simulink model "RadarSimulinkProjectRev005"  (R2024a)
settings: Solver=VariableStepAuto  StartTime=0.0  StopTime=0.0576  RelTol=1e-3
values from neighbouring files (symbols this model uses):
  AngleTime = SweepTime/10    (= 10000)    [InitializationOfVariablesRev000.m]    (also in InitializationOfVariablesRev001.m; InitializationOfVariablesRev002.m = 2000; InitializationOfVariablesRev003.m = 20000; InitializationOfVariablesRev004.m = 2097152)
  ASR_LUT = Rsamp    [InitializationOfVariablesRev003.m]    (also in InitializationOfVariablesRev004.m = round((R*2*SystemFs)/c); InitializationOfVariablesRev005.m = round((R*2*SystemFs)/c))
  Btn_Debounce = 20000    [InitializationOfVariablesRev003.m]    (also in InitializationOfVariablesRev004.m; InitializationOfVariablesRev005.m)
  ChirpNc = 128    [InitializationOfVariablesRev004.m]    (also in InitializationOfVariablesRev005.m)
  ChirpSizeLength = length(FCW)    [InitializationOfVariablesRev004.m]    (also in InitializationOfVariablesRev005.m = 16384)
  FCW = [FCW_p1, FCW_p2]    [InitializationOfVariablesRev002.m]    (also in InitializationOfVariablesRev003.m; InitializationOfVariablesRev004.m = interp1(1:length(FCW_base), FCW_base,      linspace(1, lengt; InitializationOfVariablesRev005.m = f / SystemFs)
  filt2divide = sum(h2_int)    [InitializationOfVariablesRev004.m]
  RXFFTLength = 4096    [InitializationOfVariablesRev003.m]    (also in InitializationOfVariablesRev004.m = 1024; InitializationOfVariablesRev005.m = 2048)
  SweepTime = 100000    [InitializationOfVariablesRev000.m]    (also in InitializationOfVariablesRev001.m; InitializationOfVariablesRev002.m = 20000; InitializationOfVariablesRev003.m = 200000; InitializationOfVariablesRev004.m = 23068672)
undefined symbols (not defined in the file or in its folder): SignalGenerationForAnalysis, Subsystem, xc7a200tfbg676
libraries: hdlBasic x350, hdlDSPIP x16, hdlUtilities x11, vmcUtilities x1
(part 2 of 4)

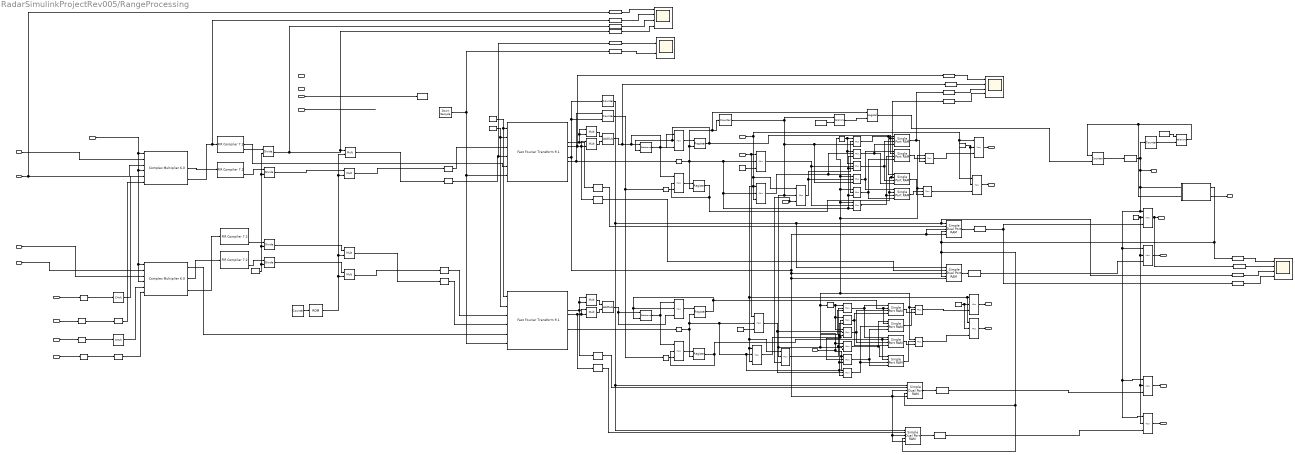
== system RadarSimulinkProjectRev005/RangeProcessing ==
  note: Tready will last until end of all 131072 samples, use for Doppler FFT
  note: These blocks are still needed for transmitting the range
  note: Will be 1 at PreDelay of EOF process, and 0 at end
      | 0 = pass through, 1 = STOP writting.
  note: Will switch to different RAM for doing the read operations, but delay not accounted
      | for the 50,000 sample delay for doppler FFT. Need to switch off WE and hold.
  note: Describes what chirp we are on, it's enable will trigger at the end of each FFT
  note: All Delays for after base Sig has been emitted
      | DDS (1) + CompMult (50) = (51)
  note: Delays per sample:
      | -Before Emittance (1)
      | -Simulated Signal (50)
      | -Recv Mixer (50)
      | -Windowing (3)
  note: TX1SimIOut
  note: TX1SimQOut
  note: TX2SimIOut
  note: TX2SimQOut
  note: TX1_REFIOut
  note: TX1_REFQOut
  note: TX2_REFIOut
  note: TX2_REFQOut
  note: Dechirp (mix with reference)
  note: Timing Assist Values (11=EOF pulse, 10=Frame Start, 9=chirp start pulse)
  note: WindowingFunction
  note: Windowing Multiplication
  note: For Syncronization: All references to frame and chirp switching need to be delayed only by the amount of delay between when it is called to toggle, and when it leaves the radar system.
      |
      | For any delay occuring within the simulation part after, this must be accounted for in the addressable shift register (delay) which simulates range delay. This delay has nothing to do with determinng when a chirp or frame has started/ended. The minimum delay, if not 0, will need to be acounted for.
      |
      | For any delay after reception, such as windowing or multiplication, this delay is relevant to anything that has to do with the processes that depend on knowing when a frame or chirp has started/ended. Since it should only start sampling once a signal theoretically should have arrived from 0 meters (no sim delay)
  note: All Delays After Dechirp
      | Delay = (101)
  note: Delay, accounting for sample missmatch
      | Delay = (104 + 139) = (243)
  note: All Delays After Window
      | Delay = (104)
  TX1SimQOut : Inport
  TX1SimIOut : Inport  Port=2
  TX2SimQOut : Inport  Port=3
  TX2SimIOut : Inport  Port=4
  TX1_REFQOut : Inport  Port=5
  TX1_REFIOut : Inport  Port=6
  TX2_REFQOut : Inport  Port=7
  TX2_REFIOut : Inport  Port=8
  BgnChirp : Inport  Port=9
  BgnFrame : Inport  Port=10
  EOChirp : Inport  Port=11
  tvalid : Inport  Port=12
  EOFDataSel : Inport  Port=13
  EOFDataAdrr : Inport  Port=14
  FlipRAM : Inport  Port=15
  PreDelayWEDisable : Inport  Port=16
  Middleofchirp : Inport  Port=17
  ADDRSwitch{,1..3} (4 alike) : hdlBasic/Mux  inputs=2  en=off  latency=0  precision=Full  arith_type=Unsigned  n_bits=16  bin_pt=14  quantization=Truncate  overflow=Wrap  XmcBlockStatus=1  maskContainerNames=tabcontainer1  block_type=mux  block_config=sysgen:Mux_config
  AddSub : hdlBasic/AddSub  mode=Addition  use_carryin=off  use_carryout=off  en=off  latency=0  precision=Full  arith_type=Unsigned  n_bits=16  bin_pt=14  quantization=Truncate  overflow=Wrap  use_behavioral_HDL=off  hw_selection=Fabric  pipelined=off  XmcBlockStatus=1  maskContainerNames=tabcontainer1  block_type=addsub  block_config=sysgen:Addsub_config
  AddSub1 : hdlBasic/AddSub  mode=Addition  use_carryin=off  use_carryout=off  en=off  latency=0  precision=Full  arith_type=Unsigned  n_bits=16  bin_pt=14  quantization=Truncate  overflow=Wrap  use_behavioral_HDL=off  hw_selection=Fabric  pipelined=off  XmcBlockStatus=1  maskContainerNames=tabcontainer1  block_type=addsub  block_config=sysgen:Addsub_config
  AddrCountPerChirp : hdlBasic/Counter  cnt_type=Count limited  cnt_to=ChirpNc-1  operation=Up  start_count=0  cnt_by_val=1  arith_type=Unsigned  n_bits=7  bin_pt=0  load_pin=off  rst=off  en=on  explicit_period=Explicit  period=P1  use_behavioral_HDL=off  implementation=Fabric  XmcBlockStatus=1  maskContainerNames=group1  block_type=counter  block_config=sysgen:Counter_config  block_width=531  block_height=1023
  AddrforIQvals : hdlBasic/Counter  cnt_type=Count limited  cnt_to=ChirpNc*RXFFTLength-1  operation=Up  start_count=0  cnt_by_val=1  arith_type=Unsigned  n_bits=17  bin_pt=0  load_pin=off  rst=off  en=on  explicit_period=Explicit  period=P1  use_behavioral_HDL=off  implementation=Fabric  XmcBlockStatus=1  maskContainerNames=group1  block_type=counter  block_config=sysgen:Counter_config  block_width=531  block_height=1023
  CMult : hdlBasic/CMult  const=-1  gui_display_data_type=Fixed-point  const_n_bits=1  const_bin_pt=0  float_type=Single  exp_bits=8  fraction_bits=24  en=off  latency=0  precision=Full  arith_type="Signed  (2's comp)"  n_bits=16  bin_pt=14  quantization=Truncate  overflow=Wrap  use_behavioral_HDL=off  mem_type=Distributed RAM  pipeline=off  XmcBlockStatus=1  maskContainerNames=tabcontainer1  block_type=cmult  block_config=sysgen:CMult_config
      settings: infoedit=[]
  CMult1 : hdlBasic/CMult  const=-1  gui_display_data_type=Fixed-point  const_n_bits=1  const_bin_pt=0  float_type=Single  exp_bits=8  fraction_bits=24  en=off  latency=0  precision=Full  arith_type="Signed  (2's comp)"  n_bits=16  bin_pt=14  quantization=Truncate  overflow=Wrap  use_behavioral_HDL=off  mem_type=Distributed RAM  pipeline=off  XmcBlockStatus=1  maskContainerNames=tabcontainer1  block_type=cmult  block_config=sysgen:CMult_config
      settings: infoedit=[]
  ChirpSamples : hdlBasic/Constant  const=ChirpNc*RXFFTLength-1  gui_display_data_type=Fixed-point  arith_type=Unsigned  n_bits=32  bin_pt=0  preci_type=Single  exp_width=8  frac_width=24  explicit_period=on  period=P2  XmcBlockStatus=1  maskContainerNames=tabcontainer1  block_type=constant  block_config=sysgen:Constant_config
  Complex Multiplier 6.0 : hdlDSPIP/Complex Multiplier 6.0   datatype=integer  hasatlast=off  hasatuser=off  atuserwidth=1  hasbtlast=off  hasbtuser=off  btuserwidth=1  multtype=Use_Mults  optimizegoal=Resources  flowcontrol=NonBlocking  outputwidth=34  roundmode=Truncate  hasctrltlast=off  hasctrltuser=off  ctrltuserwidth=1  outtlastbehv=Null  latencyconfig=Manual  minimumlatency=50  aclken=off  aresetn=off  trim_axipin_name=on  simulation_type=hybrid_sim  simulation_model=sysgen:cmpy_v6_0  data_path_portlist={ 's_axis_a_tdata_real', 's_axis_a_tdata_imag', 's_axis_b_tdata_real', 's_axis_b_tdata_imag', 's_axis_ctrl_tdata_rounding_bit', 'm_axis_dout_tdata_real', 'm_axis_dout_tdata_imag' }  aportwidth=63  bportwidth=63  ip_name=Complex Multiplier  ip_version=6.0  dsptool_ready=true  ipcore_usecache=true  ipcore_useipmodelcache=true  ipcore_verbose=false  ipcore_latency_parameter='minimumlatency'  wrapper_available=true  port_translation_map={ 'aclken' => 'en', 'aresetn' => 'rst'}  XmcBlockStatus=1  maskContainerNames=tabcontainer1  block_type=cmpy_v6_0  block_config=sysgen:rodinimport_config
  Complex Multiplier 6.1 : hdlDSPIP/Complex Multiplier 6.0   datatype=integer  hasatlast=off  hasatuser=off  atuserwidth=1  hasbtlast=off  hasbtuser=off  btuserwidth=1  multtype=Use_Mults  optimizegoal=Resources  flowcontrol=NonBlocking  outputwidth=34  roundmode=Truncate  hasctrltlast=off  hasctrltuser=off  ctrltuserwidth=1  outtlastbehv=Null  latencyconfig=Manual  minimumlatency=50  aclken=off  aresetn=off  trim_axipin_name=on  simulation_type=hybrid_sim  simulation_model=sysgen:cmpy_v6_0  data_path_portlist={ 's_axis_a_tdata_real', 's_axis_a_tdata_imag', 's_axis_b_tdata_real', 's_axis_b_tdata_imag', 's_axis_ctrl_tdata_rounding_bit', 'm_axis_dout_tdata_real', 'm_axis_dout_tdata_imag' }  aportwidth=63  bportwidth=63  ip_name=Complex Multiplier  ip_version=6.0  dsptool_ready=true  ipcore_usecache=true  ipcore_useipmodelcache=true  ipcore_verbose=false  ipcore_latency_parameter='minimumlatency'  wrapper_available=true  port_translation_map={ 'aclken' => 'en', 'aresetn' => 'rst'}  XmcBlockStatus=1  maskContainerNames=tabcontainer1  block_type=cmpy_v6_0  block_config=sysgen:rodinimport_config
  Constant : hdlBasic/Constant  const=filt2divide  gui_display_data_type=Fixed-point  arith_type=Signed (2's comp)  n_bits=32  bin_pt=0  preci_type=Single  exp_width=8  frac_width=24  explicit_period=off  period=1/200e6  XmcBlockStatus=1  maskContainerNames=tabcontainer1  block_type=constant  block_config=sysgen:Constant_config
  Constant2 : hdlBasic/Constant  const=0  gui_display_data_type=Fixed-point  arith_type=Signed (2's comp)  n_bits=16  bin_pt=15  preci_type=Single  exp_width=8  frac_width=24  explicit_period=on  period=P2  XmcBlockStatus=1  maskContainerNames=tabcontainer1  block_type=constant  block_config=sysgen:Constant_config
  Constant4 : hdlBasic/Constant  const=0  gui_display_data_type=Boolean  arith_type=Boolean  n_bits=16  bin_pt=15  preci_type=Single  exp_width=8  frac_width=24  explicit_period=on  period=P2  XmcBlockStatus=1  maskContainerNames=tabcontainer1  block_type=constant  block_config=sysgen:Constant_config
  Constant5 : hdlBasic/Constant  const=0  gui_display_data_type=Boolean  arith_type=Boolean  n_bits=16  bin_pt=15  preci_type=Single  exp_width=8  frac_width=24  explicit_period=on  period=P2  XmcBlockStatus=1  maskContainerNames=tabcontainer1  block_type=constant  block_config=sysgen:Constant_config
  Constant6 : hdlBasic/Constant  const=0  gui_display_data_type=Fixed-point  arith_type=Signed (2's comp)  n_bits=16  bin_pt=15  preci_type=Single  exp_width=8  frac_width=24  explicit_period=on  period=P2  XmcBlockStatus=1  maskContainerNames=tabcontainer1  block_type=constant  block_config=sysgen:Constant_config
  Constant7 : hdlBasic/Constant  const=0  gui_display_data_type=Fixed-point  arith_type=Signed (2's comp)  n_bits=16  bin_pt=15  preci_type=Single  exp_width=8  frac_width=24  explicit_period=on  period=P2  XmcBlockStatus=1  maskContainerNames=tabcontainer1  block_type=constant  block_config=sysgen:Constant_config
  Convert : hdlBasic/Convert  gui_display_data_type=Fixed-point  arith_type=Signed (2's comp)  n_bits=17  bin_pt=15  float_type=Single  exp_bits=8  fraction_bits=24  quantization=Truncate  overflow=Wrap  en=off  latency=0  pipeline=off  XmcBlockStatus=1  maskContainerNames=group2  block_type=convert  block_config=sysgen:Convert_config  block_width=595  block_height=885
  Convert1 : hdlBasic/Convert  gui_display_data_type=Fixed-point  arith_type=Signed (2's comp)  n_bits=17  bin_pt=15  float_type=Single  exp_bits=8  fraction_bits=24  quantization=Truncate  overflow=Wrap  en=off  latency=0  pipeline=off  XmcBlockStatus=1  maskContainerNames=group2  block_type=convert  block_config=sysgen:Convert_config  block_width=595  block_height=885
  Convert{7..10} (4 alike) : hdlBasic/Convert  gui_display_data_type=Fixed-point  arith_type=Signed (2's comp)  n_bits=17  bin_pt=16  float_type=Single  exp_bits=8  fraction_bits=24  quantization=Truncate  overflow=Saturate  en=off  latency=0  pipeline=off  XmcBlockStatus=1  maskContainerNames=group2  block_type=convert  block_config=sysgen:Convert_config  block_width=595  block_height=885
  Convert{2..5} (4 alike) : hdlBasic/Convert  gui_display_data_type=Fixed-point  arith_type=Signed (2's comp)  n_bits=16  bin_pt=15  float_type=Single  exp_bits=8  fraction_bits=24  quantization="Round  (unbiased: +/- Inf)"  overflow=Saturate  en=off  latency=0  pipeline=off  XmcBlockStatus=1  maskContainerNames=group2  block_type=convert  block_config=sysgen:Convert_config  block_width=595  block_height=885
  Convert6 : hdlBasic/Convert  gui_display_data_type=Boolean  arith_type=Boolean  n_bits=16  bin_pt=14  float_type=Single  exp_bits=8  fraction_bits=24  quantization=Truncate  overflow=Wrap  en=off  latency=0  pipeline=off  XmcBlockStatus=1  maskContainerNames=group2  block_type=convert  block_config=sysgen:Convert_config  block_width=595  block_height=885
  Counter : hdlBasic/Counter  cnt_type=Count limited  cnt_to=1  operation=Up  start_count=0  cnt_by_val=1  arith_type=Unsigned  n_bits=1  bin_pt=0  load_pin=off  rst=on  en=on  explicit_period=Explicit  period=P1  use_behavioral_HDL=off  implementation=Fabric  XmcBlockStatus=1  maskContainerNames=group1  block_type=counter  block_config=sysgen:Counter_config  block_width=531  block_height=1023
  Counter2 : hdlBasic/Counter  cnt_type=Count limited  cnt_to=(ChirpNc*RXFFTLength)-1  operation=Up  start_count=0  cnt_by_val=1  arith_type=Unsigned  n_bits=17  bin_pt=0  load_pin=off  rst=off  en=on  explicit_period=Explicit  period=P1  use_behavioral_HDL=off  implementation=Fabric  XmcBlockStatus=1  maskContainerNames=group1  block_type=counter  block_config=sysgen:Counter_config  block_width=531  block_height=1023
  Delay{1,12..16} (6 alike) : hdlBasic/Delay  rst=off  en=off  latency=3  reg_retiming=off  XmcBlockStatus=1  maskContainerNames=group1  block_type=delay  block_config=sysgen:Delay_config
  Delay11 : hdlBasic/Delay  rst=off  en=off  latency=104  reg_retiming=off  XmcBlockStatus=1  maskContainerNames=group1  block_type=delay  block_config=sysgen:Delay_config
  Delay17 : hdlBasic/Delay  rst=off  en=off  latency=1  reg_retiming=off  XmcBlockStatus=1  maskContainerNames=group1  block_type=delay  block_config=sysgen:Delay_config
  Delay2 : hdlBasic/Delay  rst=off  en=off  latency=1  reg_retiming=off  XmcBlockStatus=1  maskContainerNames=group1  block_type=delay  block_config=sysgen:Delay_config
  Down Sample : hdlBasic/Down Sample  sample_ratio=16  sample_phase="Last Value of Frame  (most efficient)"  en=off  rst=off  latency=1  XmcBlockStatus=1  maskContainerNames=group1  block_type=dsamp  block_config=sysgen:Downsample_config
  ENSwitch{,1..3} (4 alike) : hdlBasic/Mux  inputs=2  en=off  latency=0  precision=Full  arith_type=Unsigned  n_bits=16  bin_pt=14  quantization=Truncate  overflow=Wrap  XmcBlockStatus=1  maskContainerNames=tabcontainer1  block_type=mux  block_config=sysgen:Mux_config
  EOFRAADDR : hdlBasic/Mux  inputs=2  en=off  latency=0  precision=Full  arith_type=Unsigned  n_bits=16  bin_pt=14  quantization=Truncate  overflow=Wrap  XmcBlockStatus=1  maskContainerNames=tabcontainer1  block_type=mux  block_config=sysgen:Mux_config
  EOFRAADDR2 : hdlBasic/Mux  inputs=2  en=off  latency=0  precision=Full  arith_type=Unsigned  n_bits=16  bin_pt=14  quantization=Truncate  overflow=Wrap  XmcBlockStatus=1  maskContainerNames=tabcontainer1  block_type=mux  block_config=sysgen:Mux_config
  EOFRAMen1 : hdlBasic/Mux  inputs=2  en=off  latency=0  precision=Full  arith_type=Unsigned  n_bits=16  bin_pt=14  quantization=Truncate  overflow=Wrap  XmcBlockStatus=1  maskContainerNames=tabcontainer1  block_type=mux  block_config=sysgen:Mux_config
  EOFRAMen3 : hdlBasic/Mux  inputs=2  en=off  latency=0  precision=Full  arith_type=Unsigned  n_bits=16  bin_pt=14  quantization=Truncate  overflow=Wrap  XmcBlockStatus=1  maskContainerNames=tabcontainer1  block_type=mux  block_config=sysgen:Mux_config
  EOFRAMwe1 : hdlBasic/Mux  inputs=2  en=off  latency=0  precision=Full  arith_type=Unsigned  n_bits=16  bin_pt=14  quantization=Truncate  overflow=Wrap  XmcBlockStatus=1  maskContainerNames=tabcontainer1  block_type=mux  block_config=sysgen:Mux_config
  EOFRAMwe2 : hdlBasic/Mux  inputs=2  en=off  latency=0  precision=Full  arith_type=Unsigned  n_bits=16  bin_pt=14  quantization=Truncate  overflow=Wrap  XmcBlockStatus=1  maskContainerNames=tabcontainer1  block_type=mux  block_config=sysgen:Mux_config
  FFTSamplingRelation : hdlBasic/Relational  mode=a=b  op_type=Bool  en=off  latency=0  XmcBlockStatus=1  maskContainerNames=tabcontainer1  block_type=relational  block_config=sysgen:Relational_config
  FFT_C1 : hdlBasic/Constant  const=1.0  gui_display_data_type=Fixed-point  arith_type=Unsigned  n_bits=1  bin_pt=0  preci_type=Single  exp_width=8  frac_width=24  explicit_period=on  period=P2  XmcBlockStatus=1  maskContainerNames=tabcontainer1  block_type=constant  block_config=sysgen:Constant_config
  FFT_C2 : hdlBasic/Constant  const=1.0  gui_display_data_type=Boolean  arith_type=Boolean  n_bits=1  bin_pt=0  preci_type=Single  exp_width=8  frac_width=24  explicit_period=on  period=P2  XmcBlockStatus=1  maskContainerNames=tabcontainer1  block_type=constant  block_config=sysgen:Constant_config
  FIR Compiler 7.{1..4} (4 alike) : hdlDSPIP/FIR Compiler 7.2   coefficientvector=h2_int  coefficient_sets=1  coefficient_reload=off  filter_type=Decimation  rate_change_type=Integer  interpolation_rate=1  decimation_rate=16  zero_pack_factor=1  channel_sequence=Basic  number_channels=1  pattern_list='P4-0,P4-1,P4-2,P4-3,P4-4'  number_paths=1  ratespecification=Maximum_Possible  sampleperiod=1  hardwareoversamplingrate=1  coefficient_sign=Unsigned  quantization=Integer_Coefficients  coefficient_width=16  bestprecision=off  coefficient_fractional_bits=0  coefficient_structure=Inferred  output_rounding_mode=Full_Precision  output_width=36  filter_architecture=Systolic_Multiply_Accumulate  optimization_goal=Area  optimization_list='None'  data_buffer_type=Automatic  coefficient_buffer_type=Automatic  input_buffer_type=Automatic  output_buffer_type=Automatic  preference_for_other_storage=Automatic  multi_column_support=Automatic  columnconfig='8'  inter_column_pipe_length=4  data_has_tlast=Not_Required  m_data_has_tready=off  s_data_has_fifo=off  s_data_has_tuser=Not_Required  m_data_has_tuser=Not_Required  s_config_sync_mode=On_Vector  s_config_method=Single  num_reload_slots=1  has_aclken=off  has_aresetn=off  reset_data_vector=on  trim_axipin_name=on  simulation_type=hybrid_sim  simulation_model=sysgen:xfirv7_2_cmodel  data_path_portlist={ 's_axis_data_tdata', 'm_axis_data_tdata' }  passband_min=0.0  passband_max=0.5  stopband_min=0.5  stopband_max=1.0  filter_selection=1  gui_behaviour='Sysgen_GUI'  data_sign=Signed  data_width=16  data_fractional_bits=0  data_tuser_width=1  wrapper_available=true  ip_wrap_arbitrary_binary_point=true  ip_name=FIR Compiler  ip_version=7.2  dsptool_ready=true  ipcore_usecache=true  ipcore_useipmodelcache=true  port_translation_map={ 'aclken' => 'en', 'aresetn' => 'rst' }  run_core_at_system_period=true  ipcore_xco_need_fpga_part=true  ipcore_fpga_part=[]  XmcBlockStatus=1  maskContainerNames=tabcontainer1  block_type=fir_compiler_v7_2  block_config=sysgen:rodinimport_config  block_width=820  block_height=600
  FIRCompensate{,1..3} (4 alike) : hdlBasic/Delay  rst=off  en=off  latency=filt_delay  reg_retiming=off  XmcBlockStatus=1  maskContainerNames=group1  block_type=delay  block_config=sysgen:Delay_config
  Fast Fourier Transform 9.1 : hdlDSPIP/Fast Fourier Transform 9.1   transform_length=1024  target_clock_frequency=250  target_data_throughput=50  implementation_options=pipelined_streaming_io  run_time_configurable_transform_length=off  enable_ssr=off  super_sample_rates=1  data_format=fixed_point  phase_factor_width=24  scaling_options=block_floating_point  rounding_modes=truncation  aclken=off  aresetn=off  output_ordering=natural_order  cyclic_prefix_insertion=off  throttle_scheme=realtime  xk_index=on  ovflo=off  trim_axipin_name=on  memory_options_data=block_ram  memory_options_phase_factors=block_ram  number_of_stages_using_block_ram_for_data_and_phase_factors=1  memory_options_reorder=block_ram  memory_options_hybrid=off  complex_mult_type=use_mults_performance  butterfly_type=use_xtremedsp_slices  simulation_type=hybrid_sim  simulation_model=sysgen:xfftv9_cmodel  data_path_portlist={ 's_axis_data_tdata', 'm_axis_data_tdata', 'm_axis_status_tdata', 'event_fft_overflow' }  channels=1  input_ordering=natural_order  input_width=16  ip_name=Fast Fourier Transform  ip_version=9.1  dsptool_ready=true  ipcore_usecache=true  ipcore_useipmodelcache=true  wrapper_available=true  port_translation_map={ 'aclken' => 'en', 'aresetn' => 'rst'}  XmcBlockStatus=1  maskContainerNames=tabcontainer1  block_type=xfft_v9_1  block_config=sysgen:rodinimport_config
  Fast Fourier Transform 9.2 : hdlDSPIP/Fast Fourier Transform 9.1   transform_length=1024  target_clock_frequency=250  target_data_throughput=50  implementation_options=pipelined_streaming_io  run_time_configurable_transform_length=off  enable_ssr=off  super_sample_rates=1  data_format=fixed_point  phase_factor_width=24  scaling_options=block_floating_point  rounding_modes=truncation  aclken=off  aresetn=off  output_ordering=natural_order  cyclic_prefix_insertion=off  throttle_scheme=realtime  xk_index=on  ovflo=off  trim_axipin_name=on  memory_options_data=block_ram  memory_options_phase_factors=block_ram  number_of_stages_using_block_ram_for_data_and_phase_factors=1  memory_options_reorder=block_ram  memory_options_hybrid=off  complex_mult_type=use_mults_performance  butterfly_type=use_xtremedsp_slices  simulation_type=hybrid_sim  simulation_model=sysgen:xfftv9_cmodel  data_path_portlist={ 's_axis_data_tdata', 'm_axis_data_tdata', 'm_axis_status_tdata', 'event_fft_overflow' }  channels=1  input_ordering=natural_order  input_width=16  ip_name=Fast Fourier Transform  ip_version=9.1  dsptool_ready=true  ipcore_usecache=true  ipcore_useipmodelcache=true  wrapper_available=true  port_translation_map={ 'aclken' => 'en', 'aresetn' => 'rst'}  XmcBlockStatus=1  maskContainerNames=tabcontainer1  block_type=xfft_v9_1  block_config=sysgen:rodinimport_config
  Gateway Out{1..14} (14 alike) : hdlBasic/Gateway Out  inherit_from_input=off  bool_to_boolean=off  hdl_port=on  rows=1  columns=1  UseAsDAC=off  DACChannel='1'  interface=None  automatic_assignment=on  address_offset=hex2dec('00')  intf_name=''  intf_description=''  timing_constraint=None  locs_specified=off  LOCs={}  io_standard={}  XmcBlockStatus=1  maskContainerNames=group4  block_type=gatewayout  block_config=sysgen:gateway_out_config  block_width_w=590  block_height_w=620  block_width=620  block_height=750
  INDXOutSwitch : hdlBasic/Mux  inputs=2  en=off  latency=0  precision=Full  arith_type=Unsigned  n_bits=16  bin_pt=14  quantization=Truncate  overflow=Wrap  XmcBlockStatus=1  maskContainerNames=tabcontainer1  block_type=mux  block_config=sysgen:Mux_config
  INDXOutSwitch1 : hdlBasic/Mux  inputs=2  en=off  latency=0  precision=Full  arith_type=Unsigned  n_bits=16  bin_pt=14  quantization=Truncate  overflow=Wrap  XmcBlockStatus=1  maskContainerNames=tabcontainer1  block_type=mux  block_config=sysgen:Mux_config
  IndexTracker : hdlBasic/Counter  cnt_type=Count limited  cnt_to=RXFFTLength-1  operation=Up  start_count=0  cnt_by_val=1  arith_type=Unsigned  n_bits=14  bin_pt=0  load_pin=off  rst=on  en=on  explicit_period=Explicit  period=P1  use_behavioral_HDL=off  implementation=Fabric  XmcBlockStatus=1  maskContainerNames=group1  block_type=counter  block_config=sysgen:Counter_config  block_width=531  block_height=1023
  Inverter : hdlBasic/Inverter  en=off  latency=0  XmcBlockStatus=1  maskContainerNames=group2  block_type=inv  block_config=sysgen:Inverter_config
  Inverter1 : hdlBasic/Inverter  en=off  latency=0  XmcBlockStatus=1  maskContainerNames=group2  block_type=inv  block_config=sysgen:Inverter_config
  LastChirp : hdlBasic/Constant  const=0  gui_display_data_type=Fixed-point  arith_type=Unsigned  n_bits=7  bin_pt=0  preci_type=Single  exp_width=8  frac_width=24  explicit_period=on  period=P2  XmcBlockStatus=1  maskContainerNames=tabcontainer1  block_type=constant  block_config=sysgen:Constant_config
  Logical : hdlBasic/Logical  logical_function=AND  inputs=2  en=off  latency=0  precision=Full  arith_type=Unsigned  n_bits=16  bin_pt=0  align_bp=on  overflow=[]  quantization=[]  XmcBlockStatus=1  maskContainerNames=tabcontainer1  block_type=logical  block_config=sysgen:Logical_config
  MAGOutSwitch : hdlBasic/Mux  inputs=2  en=off  latency=0  precision=Full  arith_type=Unsigned  n_bits=16  bin_pt=14  quantization=Truncate  overflow=Wrap  XmcBlockStatus=1  maskContainerNames=tabcontainer1  block_type=mux  block_config=sysgen:Mux_config
  MAGOutSwitch1 : hdlBasic/Mux  inputs=2  en=off  latency=0  precision=Full  arith_type=Unsigned  n_bits=16  bin_pt=14  quantization=Truncate  overflow=Wrap  XmcBlockStatus=1  maskContainerNames=tabcontainer1  block_type=mux  block_config=sysgen:Mux_config
  Mult{4..7} (4 alike) : hdlBasic/Mult  precision=Full  arith_type="Signed  (2's comp)"  n_bits=16  bin_pt=14  quantization=Truncate  overflow=Wrap  en=off  latency=3  opt_float=off  fp_mult_usage=No Usage  use_behavioral_HDL=off  opt=Speed  use_embedded=on  optimum_pipeline=off  pipeline=on  use_rpm=on  placement_style=Triangular  XmcBlockStatus=1  maskContainerNames=group1  block_type=mult  block_config=sysgen:Mult_config  block_width=598  block_height=876
  Mux{,1,6..7,12..19} (12 alike) : hdlBasic/Mux  inputs=2  en=off  latency=0  precision=Full  arith_type=Unsigned  n_bits=16  bin_pt=14  quantization=Truncate  overflow=Wrap  XmcBlockStatus=1  maskContainerNames=tabcontainer1  block_type=mux  block_config=sysgen:Mux_config
  PeakAmp RAM{1..4} (4 alike) : hdlBasic/Single Port RAM  depth=ChirpNc  initVector=0  distributed_mem=Block RAM  write_mode=Read After Write  rst=off  init_reg=0  en=on  optimize_latency=off  latency=1  optimize=Area  dbl_ovrd=off  simulation_type=fast_sim  XmcBlockStatus=1  maskContainerNames=tabcontainer1  block_type=spram  block_config=sysgen:SPRAM_config
  PeakAmplitude1 : hdlBasic/Register  init=0  rst=on  en=off  XmcBlockStatus=1  maskContainerNames=tabcontainer1  block_type=register  block_config=sysgen:Register_config
  PeakAmplitude2 : hdlBasic/Register  init=0  rst=on  en=off  XmcBlockStatus=1  maskContainerNames=tabcontainer1  block_type=register  block_config=sysgen:Register_config
  PeakIndex1 : hdlBasic/Register  init=0  rst=on  en=off  XmcBlockStatus=1  maskContainerNames=tabcontainer1  block_type=register  block_config=sysgen:Register_config
  PeakIndex2 : hdlBasic/Register  init=0  rst=on  en=off  XmcBlockStatus=1  maskContainerNames=tabcontainer1  block_type=register  block_config=sysgen:Register_config
  PeakIndx RAM{1..4} (4 alike) : hdlBasic/Single Port RAM  depth=ChirpNc  initVector=0  distributed_mem=Block RAM  write_mode=Read After Write  rst=off  init_reg=0  en=on  optimize_latency=off  latency=1  optimize=Area  dbl_ovrd=off  simulation_type=fast_sim  XmcBlockStatus=1  maskContainerNames=tabcontainer1  block_type=spram  block_config=sysgen:SPRAM_config
  Q1 : hdlBasic/Divide  flow_control=NonBlocking  axi_optimize_goal=Resources  algorithm_type=Radix2  fractional_width=16  latency=0  rate=1  has_a_tlast=off  has_a_tuser=off  has_b_tlast=off  has_b_tuser=off  en=off  has_result_tready=off  result_tlast_behv=Pass_A_TLAST  has_underflow=off  has_overflow=off  has_invalid_op=off  has_divide_by_zero=off  fpo_op_type=mergeddivide  XmcBlockStatus=1  maskContainerNames=tabcontainer1  block_type=divide  block_config=sysgen:FPOBlockDescriptor_config
  Q2 : hdlBasic/Divide  flow_control=NonBlocking  axi_optimize_goal=Resources  algorithm_type=Radix2  fractional_width=16  latency=0  rate=1  has_a_tlast=off  has_a_tuser=off  has_b_tlast=off  has_b_tuser=off  en=off  has_result_tready=off  result_tlast_behv=Pass_A_TLAST  has_underflow=off  has_overflow=off  has_invalid_op=off  has_divide_by_zero=off  fpo_op_type=mergeddivide  XmcBlockStatus=1  maskContainerNames=tabcontainer1  block_type=divide  block_config=sysgen:FPOBlockDescriptor_config
  ROM : hdlBasic/ROM  depth=ChirpSizeLength/16  initVector=WindowCoefficients  distributed_mem=Block RAM  rst=off  init_reg=0  en=off  latency=1  gui_display_data_type=Fixed-point  arith_type=Unsigned  n_bits=16  bin_pt=16  preci_type=Single  exp_width=8  frac_width=24  optimize=Area  use_rpm=on  simulation_type=fast_sim  XmcBlockStatus=1  maskContainerNames=tabcontainer1  block_type=sprom  block_config=sysgen:SPROM_config
  Re1 : hdlBasic/Divide  flow_control=NonBlocking  axi_optimize_goal=Resources  algorithm_type=Radix2  fractional_width=16  latency=0  rate=1  has_a_tlast=off  has_a_tuser=off  has_b_tlast=off  has_b_tuser=off  en=off  has_result_tready=off  result_tlast_behv=Pass_A_TLAST  has_underflow=off  has_overflow=off  has_invalid_op=off  has_divide_by_zero=off  fpo_op_type=mergeddivide  XmcBlockStatus=1  maskContainerNames=tabcontainer1  block_type=divide  block_config=sysgen:FPOBlockDescriptor_config
  Re2 : hdlBasic/Divide  flow_control=NonBlocking  axi_optimize_goal=Resources  algorithm_type=Radix2  fractional_width=16  latency=0  rate=1  has_a_tlast=off  has_a_tuser=off  has_b_tlast=off  has_b_tuser=off  en=off  has_result_tready=off  result_tlast_behv=Pass_A_TLAST  has_underflow=off  has_overflow=off  has_invalid_op=off  has_divide_by_zero=off  fpo_op_type=mergeddivide  XmcBlockStatus=1  maskContainerNames=tabcontainer1  block_type=divide  block_config=sysgen:FPOBlockDescriptor_config
  Relational : hdlBasic/Relational  mode=a>b  op_type=Bool  en=off  latency=0  XmcBlockStatus=1  maskContainerNames=tabcontainer1  block_type=relational  block_config=sysgen:Relational_config
  Relational2 : hdlBasic/Relational  mode=a>b  op_type=Bool  en=off  latency=0  XmcBlockStatus=1  maskContainerNames=tabcontainer1  block_type=relational  block_config=sysgen:Relational_config
  Scope1 : Scope  NumInputPorts=4
  Scope2 : Scope  NumInputPorts=4
  Scope3 : Scope  NumInputPorts=2
  Scope4 : Scope  NumInputPorts=4
  Simple Dual Port RAM{,1..3} (4 alike) : hdlBasic/Simple Dual Port RAM  depth=ChirpNc*RXFFTLength  initVector=0  distributed_mem=Distributed memory  init_b=0  rst_b=off  en_a=on  en_b=off  latency=1  write_mode_B=Read After Write  explicit_period=[]  period=[]  simulation_type=fast_sim  XmcBlockStatus=1  maskContainerNames=tabcontainer1  block_type=sdpram  block_config=sysgen:Sdpram_config  optimize=Area
      settings: infoedit=[]
  Subsystem : Subsystem
  TlastChirpRelation : hdlBasic/Relational  mode=a=b  op_type=Bool  en=off  latency=0  XmcBlockStatus=1  maskContainerNames=tabcontainer1  block_type=relational  block_config=sysgen:Relational_config
  WeSwitch{1..4} (4 alike) : hdlBasic/Mux  inputs=2  en=off  latency=0  precision=Full  arith_type=Unsigned  n_bits=16  bin_pt=14  quantization=Truncate  overflow=Wrap  XmcBlockStatus=1  maskContainerNames=tabcontainer1  block_type=mux  block_config=sysgen:Mux_config
  WinImag1 : hdlBasic/Mult  precision=Full  arith_type="Signed  (2's comp)"  n_bits=16  bin_pt=14  quantization=Truncate  overflow=Wrap  en=off  latency=0  opt_float=off  fp_mult_usage=No Usage  use_behavioral_HDL=off  opt=Speed  use_embedded=on  optimum_pipeline=off  pipeline=on  use_rpm=on  placement_style=Triangular  XmcBlockStatus=1  maskContainerNames=group1  block_type=mult  block_config=sysgen:Mult_config  block_width=598  block_height=876
  WinImag2 : hdlBasic/Mult  precision=Full  arith_type="Signed  (2's comp)"  n_bits=16  bin_pt=14  quantization=Truncate  overflow=Wrap  en=off  latency=0  opt_float=off  fp_mult_usage=No Usage  use_behavioral_HDL=off  opt=Speed  use_embedded=on  optimum_pipeline=off  pipeline=on  use_rpm=on  placement_style=Triangular  XmcBlockStatus=1  maskContainerNames=group1  block_type=mult  block_config=sysgen:Mult_config  block_width=598  block_height=876
  WinReal1 : hdlBasic/Mult  precision=Full  arith_type="Signed  (2's comp)"  n_bits=16  bin_pt=14  quantization=Truncate  overflow=Wrap  en=off  latency=0  opt_float=off  fp_mult_usage=No Usage  use_behavioral_HDL=off  opt=Speed  use_embedded=on  optimum_pipeline=off  pipeline=on  use_rpm=on  placement_style=Triangular  XmcBlockStatus=1  maskContainerNames=group1  block_type=mult  block_config=sysgen:Mult_config  block_width=598  block_height=876
  WinReal2 : hdlBasic/Mult  precision=Full  arith_type="Signed  (2's comp)"  n_bits=16  bin_pt=14  quantization=Truncate  overflow=Wrap  en=off  latency=0  opt_float=off  fp_mult_usage=No Usage  use_behavioral_HDL=off  opt=Speed  use_embedded=on  optimum_pipeline=off  pipeline=on  use_rpm=on  placement_style=Triangular  XmcBlockStatus=1  maskContainerNames=group1  block_type=mult  block_config=sysgen:Mult_config  block_width=598  block_height=876
  WindowPeriod : hdlBasic/Counter  cnt_type=Count limited  cnt_to=(ChirpSizeLength/16)-1  operation=Up  start_count=0  cnt_by_val=1  arith_type=Unsigned  n_bits=10  bin_pt=0  load_pin=off  rst=off  en=off  explicit_period=Explicit  period=P2  use_behavioral_HDL=off  implementation=Fabric  XmcBlockStatus=1  maskContainerNames=group1  block_type=counter  block_config=sysgen:Counter_config  block_width=531  block_height=1023
  RngImagTx1 : Outport
  RngReTx1 : Outport  Port=2
  RngImagTx2 : Outport  Port=3
  RngReTx2 : Outport  Port=4
  TlastVel : Outport  Port=5
  TreadyVel : Outport  Port=6
  EOFDataMAG1 : Outport  Port=7
  EOFDataIDX1 : Outport  Port=8
  EOFDataMAG2 : Outport  Port=9
  EOFDataIDX2 : Outport  Port=10
  wires:
  WindowPeriod/1 -> ROM/1
  BgnChirp/1 -> ?
  FFT_C1/1 -> Fast Fourier Transform 9.2/1, Fast Fourier Transform 9.1/1
  CMult1/1 -> Complex Multiplier 6.0/5
  Convert1/1 -> Complex Multiplier 6.0/6
  CMult/1 -> Complex Multiplier 6.1/5
  Convert/1 -> Complex Multiplier 6.1/6
  Complex Multiplier 6.1/2 -> FIR Compiler 7.4/1  "TX2Q"
  Complex Multiplier 6.1/3 -> FIR Compiler 7.3/1  "TX2I"
  TX1_REFQOut/1 -> FIRCompensate/1
  TX1_REFIOut/1 -> FIRCompensate1/1
  TX2_REFQOut/1 -> FIRCompensate2/1
  TX2_REFIOut/1 -> FIRCompensate3/1
  BgnFrame/1 -> Delay11/1
  FFT_C2/1 -> Fast Fourier Transform 9.1/2, Fast Fourier Transform 9.2/2
  PeakAmplitude1/1 -> Relational/2, Mux/2, PeakAmp RAM4/2, PeakAmp RAM1/2
  Mux/1 -> PeakAmplitude1/1
  Mux1/1 -> PeakIndex1/1
  Fast Fourier Transform 9.1/10 -> Delay2/1, IndexTracker/1
  Fast Fourier Transform 9.1/9 -> AddrforIQvals/1, IndexTracker/2, Simple Dual Port RAM3/3, Simple Dual Port RAM3/5, Simple Dual Port RAM2/3, Simple Dual Port RAM2/5, Simple Dual Port RAM1/5, Simple Dual Port RAM1/3, Simple Dual Port RAM/5, Simple Dual Port RAM/3
  Delay1/1 -> Mux1/3
  PeakIndex1/1 -> Gateway Out10/1, PeakIndx RAM1/2, PeakIndx RAM4/2, Mux1/2
  Gateway Out10/1 -> Scope2/4
  Gateway Out9/1 -> Scope2/3
  Gateway Out7/1 -> Scope2/1
  Gateway Out8/1 -> Scope2/2
  Convert5/1 -> Fast Fourier Transform 9.1/3
  Convert3/1 -> Gateway Out4/1, Fast Fourier Transform 9.1/4
  tvalid/1 -> Complex Multiplier 6.1/4, Complex Multiplier 6.1/1, Complex Multiplier 6.0/4, Complex Multiplier 6.0/1
  ROM/1 -> WinReal1/2, WinImag1/2, WinReal2/2, WinImag2/2
  AddSub/1 -> Gateway Out8/1, Relational/1, Mux/3
  Mult5/1 -> AddSub/1
  Mult4/1 -> AddSub/2
  Complex Multiplier 6.0/3 -> Gateway Out3/1, FIR Compiler 7.2/1
  Delay13/1 -> Simple Dual Port RAM/2
  Relational/1 -> Mux1/1, Mux/1
  Delay12/1 -> Simple Dual Port RAM1/2
  Relational2/1 -> Mux7/1, Mux6/1
  IndexTracker/1 -> Delay14/1, Delay1/1
  Fast Fourier Transform 9.2/5 -> Delay16/1, Mult7/1, Mult7/2
  Mult6/1 -> AddSub1/2
  Mult7/1 -> AddSub1/1
  Delay17/1 -> EOFRAMen3/2, WeSwitch4/3, ENSwitch1/3, ENSwitch/3, WeSwitch1/3, EOFRAMwe2/2, PeakAmplitude2/2, PeakIndex2/2
  Fast Fourier Transform 9.2/6 -> Delay15/1, Mult6/1, Mult6/2
  Fast Fourier Transform 9.2/10 -> Delay17/1
  Mux7/1 -> PeakIndex2/1
  AddSub1/1 -> Mux6/3, Relational2/1
  Mux6/1 -> PeakAmplitude2/1
  PeakAmplitude2/1 -> PeakAmp RAM3/2, PeakAmp RAM2/2, Relational2/2, Mux6/2
  Delay14/1 -> Mux7/3
  Complex Multiplier 6.1/1 -> Fast Fourier Transform 9.2/5
  Convert4/1 -> Fast Fourier Transform 9.2/3
  Convert2/1 -> Fast Fourier Transform 9.2/4
  Simple Dual Port RAM2/1 -> Convert9/1  "ImagVal2"
  Simple Dual Port RAM3/1 -> Convert10/1  "ReVal2"
  LastChirp/1 -> TlastChirpRelation/2
  Convert8/1 -> Mux13/3
  Convert7/1 -> Mux12/3, Gateway Out11/1
  Logical/1 -> Counter/2  "TLast"
  TlastChirpRelation/1 -> Logical/2  "TLast"
  Counter/1 -> Convert6/1
  Counter2/1 -> FFTSamplingRelation/2
  ChirpSamples/1 -> FFTSamplingRelation/1
  FFTSamplingRelation/1 -> Counter/1, Subsystem/2(Reset)  "TLast"
  Mux12/1 -> Gateway Out13/1, RngImagTx1/1
  Mux13/1 -> RngReTx1/1
  Constant2/1 -> Mux14/2, Mux15/2, Mux13/2, Mux12/2
  Convert6/1 -> Counter2/1, TreadyVel/1, Subsystem/1(tvalid), Mux14/1, Mux15/1, Mux13/1, Mux12/1
  Convert9/1 -> Mux14/3
  Convert10/1 -> Mux15/3
  Mux14/1 -> RngImagTx2/1
  EOFRAMwe1/1 -> WeSwitch3/2, WeSwitch2/2
  EOFRAMen1/1 -> ENSwitch3/2, ENSwitch2/2
  Constant4/1 -> EOFRAMwe1/3
  EOFRAADDR2/1 -> ADDRSwitch3/2, ADDRSwitch2/2
  Mux15/1 -> RngReTx2/1
  PeakAmp RAM2/1 -> MAGOutSwitch/3  "MAGPeak2"
  PeakIndx RAM2/1 -> INDXOutSwitch/3
  EOFDataAdrr/1 -> EOFRAADDR/3, EOFRAADDR2/3
  EOFRAADDR/1 -> ADDRSwitch1/2, ADDRSwitch/2
  AddrCountPerChirp/1 -> EOFRAADDR/2, ADDRSwitch1/3, ADDRSwitch/3, EOFRAADDR2/2, ADDRSwitch2/3, ADDRSwitch3/3, TlastChirpRelation/1
  EOFRAMen3/1 -> ENSwitch/2, ENSwitch1/2
  EOFRAMwe2/1 -> WeSwitch4/2, WeSwitch1/2
  Constant5/1 -> EOFRAMwe2/3
  INDXOutSwitch1/1 -> Mux17/3
  PeakIndx RAM1/1 -> INDXOutSwitch1/3  "PeakIndx1"
  MAGOutSwitch1/1 -> Mux16/3
  PeakAmp RAM1/1 -> Gateway Out9/1, MAGOutSwitch1/3  "MAGPeak1"
  Constant6/1 -> Mux17/2, Mux16/2
  Mux16/1 -> EOFDataMAG1/1
  Mux17/1 -> EOFDataIDX1/1
  INDXOutSwitch/1 -> Mux19/3
  EOFDataSel/1 -> EOFRAADDR2/1, EOFRAADDR/1, EOFRAMen3/3, EOFRAMen3/1, Mux18/1, Mux19/1, EOFRAMen1/3, EOFRAMen1/1, Mux16/1, Mux17/1
  Constant7/1 -> Mux18/2, Mux19/2
  MAGOutSwitch/1 -> Mux18/3
  Mux19/1 -> EOFDataIDX2/1
  PeakIndex2/1 -> PeakIndx RAM3/2, PeakIndx RAM2/2, Mux7/2
  Inverter/1 -> WeSwitch4/1, ENSwitch1/1, ADDRSwitch1/1
  Inverter1/1 -> WeSwitch3/1, ENSwitch3/1, ADDRSwitch3/1
  FlipRAM/1 -> WeSwitch1/1, ENSwitch/1, Inverter1/1, ADDRSwitch2/1, ENSwitch2/1, WeSwitch2/1, INDXOutSwitch1/1, MAGOutSwitch1/1, INDXOutSwitch/1, MAGOutSwitch/1, Inverter/1, ADDRSwitch/1
  ENSwitch/1 -> PeakIndx RAM3/4, PeakAmp RAM3/4
  WeSwitch1/1 -> PeakAmp RAM3/3, PeakIndx RAM3/3
  ADDRSwitch/1 -> PeakAmp RAM3/1, PeakIndx RAM3/1
  WeSwitch4/1 -> PeakIndx RAM2/3, PeakAmp RAM2/3
  ENSwitch1/1 -> PeakIndx RAM2/4, PeakAmp RAM2/4
  ADDRSwitch1/1 -> PeakIndx RAM2/1, PeakAmp RAM2/1
  Mux18/1 -> EOFDataMAG2/1
  PeakAmp RAM3/1 -> MAGOutSwitch/2  "MAGPeak2"
  PeakIndx RAM3/1 -> INDXOutSwitch/2  "Peakindx2"
  ENSwitch2/1 -> PeakAmp RAM4/4, PeakIndx RAM4/4
  ADDRSwitch2/1 -> PeakAmp RAM4/1, PeakIndx RAM4/1
  WeSwitch3/1 -> PeakIndx RAM1/3, PeakAmp RAM1/3
  ENSwitch3/1 -> PeakIndx RAM1/4, PeakAmp RAM1/4
  ADDRSwitch3/1 -> PeakIndx RAM1/1, PeakAmp RAM1/1
  PeakAmp RAM4/1 -> MAGOutSwitch1/2  "MAGPeak2"
  PeakIndx RAM4/1 -> INDXOutSwitch1/2  "Peakindx2"
  WeSwitch2/1 -> PeakAmp RAM4/3, PeakIndx RAM4/3
  PreDelayWEDisable/1 -> EOFRAMwe2/1, EOFRAMwe1/1
  WinReal2/1 -> Convert2/1
  WinImag2/1 -> Convert4/1
  WinReal1/1 -> Convert3/1
  WinImag1/1 -> Convert5/1
  Delay2/1 -> WeSwitch2/3, ENSwitch2/3, ENSwitch3/3, WeSwitch3/3, EOFRAMen1/2, EOFRAMwe1/2, PeakAmplitude1/2, AddrCountPerChirp/1, Logical/1, PeakIndex1/2
  Fast Fourier Transform 9.1/6 -> Gateway Out7/1, Mult4/2, Mult4/1, Delay12/1
  Gateway Out1/1 -> Scope3/2
  Gateway Out3/1 -> Scope1/2
  Gateway Out4/1 -> Scope3/1
  Gateway Out2/1 -> Scope1/1
  Constant/1 -> Q1/2, Re1/2, Re2/2, Q2/2
  TX1SimQOut/1 -> Complex Multiplier 6.0/2
  TX1SimIOut/1 -> Complex Multiplier 6.0/3, Gateway Out2/1
  TX2SimQOut/1 -> Complex Multiplier 6.1/2
  TX2SimIOut/1 -> Complex Multiplier 6.1/3
  FIRCompensate/1 -> CMult1/1
  FIRCompensate1/1 -> Convert1/1
  FIRCompensate2/1 -> CMult/1
  FIRCompensate3/1 -> Convert/1
  Gateway Out6/1 -> Scope1/3
  FIR Compiler 7.2/3 -> Q1/1
  FIR Compiler 7.4/3 -> Q2/1
  FIR Compiler 7.3/3 -> Re2/1
  FIR Compiler 7.1/3 -> Re1/1
  Re2/1 -> WinReal2/1
  Q2/1 -> WinImag2/1
  Complex Multiplier 6.0/2 -> FIR Compiler 7.1/1
  Gateway Out5/1 -> Scope1/4
  AddrforIQvals/1 -> Simple Dual Port RAM3/1, Simple Dual Port RAM2/1, Simple Dual Port RAM1/1, Gateway Out14/1, Simple Dual Port RAM/1
  Simple Dual Port RAM1/1 -> Convert8/1
  Simple Dual Port RAM/1 -> Convert7/1
  Subsystem/1(AddrOut) -> Gateway Out12/1, Simple Dual Port RAM1/4, Simple Dual Port RAM3/4, Simple Dual Port RAM2/4, Simple Dual Port RAM/4
  Delay16/1 -> Simple Dual Port RAM2/2
  Delay15/1 -> Simple Dual Port RAM3/2
  Gateway Out12/1 -> Scope4/1
  Gateway Out11/1 -> Scope4/4
  Gateway Out13/1 -> Scope4/2
  Gateway Out14/1 -> Scope4/3
  Subsystem/2(FFTtlast) -> TlastVel/1
  Fast Fourier Transform 9.1/5 -> Delay13/1, Mult5/2, Mult5/1
  FIR Compiler 7.2/2 -> Fast Fourier Transform 9.1/5
  Q1/1 -> WinReal1/1, Gateway Out5/1, Gateway Out6/1
  Re1/1 -> WinImag1/1
  Down Sample/1 -> Gateway Out1/1, Fast Fourier Transform 9.2/6, Fast Fourier Transform 9.1/6
